simulink model "adc16x250_8"  (R2016b)
settings: Solver=VariableStepAuto  StartTime=0.0  StopTime=10.0  RelTol=1e-3
libraries: xbsIndex_r4 x16
settings Model: Creator=qwerty40  LastModifiedBy=qwerty40

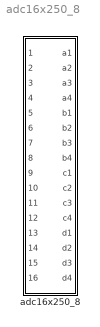
== system adc16x250_8 ==
  adc16x250_8 : Subsystem  Tag=xps:adc16  mask(ADC16){board_count=1, roach2_rev=2, zdok_rev=2}
      mask prompts: board_count "Number of ADC16 Boards"; roach2_rev "ROACH2 Revision"; zdok_rev "ZDOK Pinout Revision"
      mask help: 16-input ADC. When using one ADC16 board, it must be in ZDOK0.
      mask init:
      | % Only board_count is needed by init function
      | adc16_init(gcb, ...
      |     'board_count', board_count);
      settings: AttributesFormatString=r2 rev%<roach2_rev>\nzdok rev%<zdok_rev>
      mask Help:
      | This is the CASPER "yellow block" for the CASPER ADC16 board.  Each ADC
      | board has four ADC chips.  Each ADC chip accepts four inputs.  The four
      | 8-bit outputs from each ADC chip are concatenated into a 32-bit signal.
      mask TypeOptions board_count: 1 | 2
      mask TypeOptions roach2_rev: 1 | 2
      mask TypeOptions zdok_rev: 1 | 2

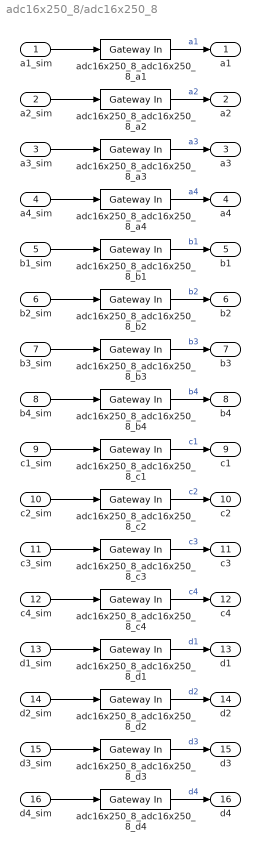
== system adc16x250_8/adc16x250_8 ==
  a1_sim : Inport
  a2_sim : Inport  Port=2
  a3_sim : Inport  Port=3
  a4_sim : Inport  Port=4
  b1_sim : Inport  Port=5
  b2_sim : Inport  Port=6
  b3_sim : Inport  Port=7
  b4_sim : Inport  Port=8
  c1_sim : Inport  Port=9
  c2_sim : Inport  Port=10
  c3_sim : Inport  Port=11
  c4_sim : Inport  Port=12
  d1_sim : Inport  Port=13
  d2_sim : Inport  Port=14
  d3_sim : Inport  Port=15
  d4_sim : Inport  Port=16
  adc16x250_8_adc16x250_8_a{1..4} (4 alike) : xbsIndex_r4/Gateway In  gui_display_data_type=Fixed-point  arith_type="Signed  (2's comp)"  n_bits=8  bin_pt=7  preci_type=Single  exp_width=8  frac_width=24  rows=1  columns=1  quantization="Round  (unbiased: +/- Inf)"  overflow=Saturate  period=1  UseAsADC=off  ADCChannel='1'  interface=None  automatic_assignment=on  address_offset=hex2dec('00')  intf_name=''  intf_description=''  default_value=0  timing_constraint=None  locs_specified=off  LOCs={}  io_standard={}  inherit_from_input=off  hdl_port=on  dbl_ovrd=off  block_type=gatewayin
  adc16x250_8_adc16x250_8_b{1..4} (4 alike) : xbsIndex_r4/Gateway In  gui_display_data_type=Fixed-point  arith_type="Signed  (2's comp)"  n_bits=8  bin_pt=7  preci_type=Single  exp_width=8  frac_width=24  rows=1  columns=1  quantization="Round  (unbiased: +/- Inf)"  overflow=Saturate  period=1  UseAsADC=off  ADCChannel='1'  interface=None  automatic_assignment=on  address_offset=hex2dec('00')  intf_name=''  intf_description=''  default_value=0  timing_constraint=None  locs_specified=off  LOCs={}  io_standard={}  inherit_from_input=off  hdl_port=on  dbl_ovrd=off  block_type=gatewayin
  adc16x250_8_adc16x250_8_c{1..4} (4 alike) : xbsIndex_r4/Gateway In  gui_display_data_type=Fixed-point  arith_type="Signed  (2's comp)"  n_bits=8  bin_pt=7  preci_type=Single  exp_width=8  frac_width=24  rows=1  columns=1  quantization="Round  (unbiased: +/- Inf)"  overflow=Saturate  period=1  UseAsADC=off  ADCChannel='1'  interface=None  automatic_assignment=on  address_offset=hex2dec('00')  intf_name=''  intf_description=''  default_value=0  timing_constraint=None  locs_specified=off  LOCs={}  io_standard={}  inherit_from_input=off  hdl_port=on  dbl_ovrd=off  block_type=gatewayin
  adc16x250_8_adc16x250_8_d{1..4} (4 alike) : xbsIndex_r4/Gateway In  gui_display_data_type=Fixed-point  arith_type="Signed  (2's comp)"  n_bits=8  bin_pt=7  preci_type=Single  exp_width=8  frac_width=24  rows=1  columns=1  quantization="Round  (unbiased: +/- Inf)"  overflow=Saturate  period=1  UseAsADC=off  ADCChannel='1'  interface=None  automatic_assignment=on  address_offset=hex2dec('00')  intf_name=''  intf_description=''  default_value=0  timing_constraint=None  locs_specified=off  LOCs={}  io_standard={}  inherit_from_input=off  hdl_port=on  dbl_ovrd=off  block_type=gatewayin
  a1 : Outport
  a2 : Outport  Port=2
  a3 : Outport  Port=3
  a4 : Outport  Port=4
  b1 : Outport  Port=5
  b2 : Outport  Port=6
  b3 : Outport  Port=7
  b4 : Outport  Port=8
  c1 : Outport  Port=9
  c2 : Outport  Port=10
  c3 : Outport  Port=11
  c4 : Outport  Port=12
  d1 : Outport  Port=13
  d2 : Outport  Port=14
  d3 : Outport  Port=15
  d4 : Outport  Port=16
  wires:
  a1_sim/1 -> adc16x250_8_adc16x250_8_a1/1
  adc16x250_8_adc16x250_8_a1/1 -> a1/1  "a1"
  a2_sim/1 -> adc16x250_8_adc16x250_8_a2/1
  adc16x250_8_adc16x250_8_a2/1 -> a2/1  "a2"
  a3_sim/1 -> adc16x250_8_adc16x250_8_a3/1
  adc16x250_8_adc16x250_8_a3/1 -> a3/1  "a3"
  a4_sim/1 -> adc16x250_8_adc16x250_8_a4/1
  adc16x250_8_adc16x250_8_a4/1 -> a4/1  "a4"
  b1_sim/1 -> adc16x250_8_adc16x250_8_b1/1
  adc16x250_8_adc16x250_8_b1/1 -> b1/1  "b1"
  b2_sim/1 -> adc16x250_8_adc16x250_8_b2/1
  adc16x250_8_adc16x250_8_b2/1 -> b2/1  "b2"
  b3_sim/1 -> adc16x250_8_adc16x250_8_b3/1
  adc16x250_8_adc16x250_8_b3/1 -> b3/1  "b3"
  b4_sim/1 -> adc16x250_8_adc16x250_8_b4/1
  adc16x250_8_adc16x250_8_b4/1 -> b4/1  "b4"
  c1_sim/1 -> adc16x250_8_adc16x250_8_c1/1
  adc16x250_8_adc16x250_8_c1/1 -> c1/1  "c1"
  c2_sim/1 -> adc16x250_8_adc16x250_8_c2/1
  adc16x250_8_adc16x250_8_c2/1 -> c2/1  "c2"
  c3_sim/1 -> adc16x250_8_adc16x250_8_c3/1
  adc16x250_8_adc16x250_8_c3/1 -> c3/1  "c3"
  c4_sim/1 -> adc16x250_8_adc16x250_8_c4/1
  adc16x250_8_adc16x250_8_c4/1 -> c4/1  "c4"
  d1_sim/1 -> adc16x250_8_adc16x250_8_d1/1
  adc16x250_8_adc16x250_8_d1/1 -> d1/1  "d1"
  d2_sim/1 -> adc16x250_8_adc16x250_8_d2/1
  adc16x250_8_adc16x250_8_d2/1 -> d2/1  "d2"
  d3_sim/1 -> adc16x250_8_adc16x250_8_d3/1
  adc16x250_8_adc16x250_8_d3/1 -> d3/1  "d3"
  d4_sim/1 -> adc16x250_8_adc16x250_8_d4/1
  adc16x250_8_adc16x250_8_d4/1 -> d4/1  "d4"
